simulink model "vco_test"  (Simulink 7.9)
settings: Solver=ode45  StartTime=0.0  StopTime=2  MaxStep=0.00001  RelTol=1e-3
values from neighbouring files (symbols this model uses):
  t_delay1 = t_delay1-0.1+0.2*rand(1)    [VCO_test.m]
  t_delay2 = t_delay2-0.1+0.2*rand(1)    [VCO_test.m]
  t_delay3 = t_delay3-0.1+0.2*rand(1)    [VCO_test.m]
libraries: dsparch4 x1, commsynccomp2 x1, commnoisgen2 x1, simulink x1, powerlib x1
settings Model: Creator=Administrator  LastModifiedBy=Administrator
settings DataIOCC: MaxDataPoints=1000000

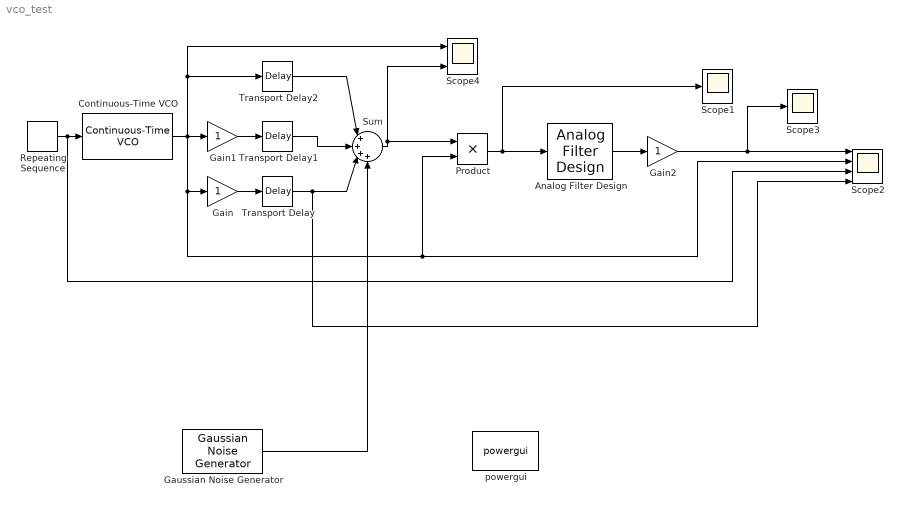
== system vco_test ==
  Analog Filter Design : dsparch4/Analog Filter Design  method=Butterworth  filttype=Lowpass  N=12  Wlo=2*3.14*25000  Whi=2*3.14*300  Rp=2  Rs=20
  Continuous-Time VCO : commsynccomp2/Continuous-Time VCO  Ac=1  Fc=100  Kc=10000  Ph=0
  Gain : Gain
  Gain1 : Gain
  Gain2 : Gain
  Gaussian Noise Generator : commnoisgen2/Gaussian Noise Generator  m=0  d=1  s=41  Ts=1  frameBased=off  sampPerFrame=1  orient=off  outDataType=double
  Product : Product  RndMeth=Zero
  Repeating Sequence : simulink/Sources/Repeating Sequence  rep_seq_t=[0 2]  rep_seq_y=[0 5]
  Scope1 : Scope
      settings: MaxDataPoints=10000001
  Scope2 : Scope  NumInputPorts=4
      settings: YMin=-5~-5~-5~-5  YMax=5~5~5~5  MaxDataPoints=131072  SampleInput=on  SampleTime=0.0001
  Scope3 : Scope
      settings: SaveName=ScopeData2  MaxDataPoints=10000001  SampleInput=on  SampleTime=0.00001
  Scope4 : Scope  NumInputPorts=2
      settings: YMin=-5~-5  YMax=5~5  SaveName=ScopeData3  MaxDataPoints=10000001  SampleInput=on  SampleTime=0.0001
  Sum : Sum  Inputs=|++++  SampleTime=0.0001
  Transport Delay : TransportDelay  DelayTime=t_delay3  BufferSize=5000000
  Transport Delay1 : TransportDelay  DelayTime=t_delay2  BufferSize=5000000
  Transport Delay2 : TransportDelay  DelayTime=t_delay1  BufferSize=5000000
  powergui : powerlib/powergui  Priority=1  SimulationMode=Discrete  SolverType=Tustin  SampleTime=1e-6  frequency=60  SPID=off  DisableSnubberDevices=off  DisableRonSwitches=off  DisableVfSwitches=off  SwTol=0  Interpol=off  DisplayEquations=off  FunctionMessages=off  frequencyindice=60  Pbase=100e6  ErrMax=1e-4  Iterations=50  UnitsV=kV  UnitsW=MW  echomessages=off  HookPort=off  EnableUseOfTLC=off  x0status=blocks  RestoreLinks=warning  ResistiveCurrentMeasurement=off  Ylog=off  Xlog=on  ShowGrid=off  save=off  variable=ZData  structure=ScopeData2  ZoomFFT=off  StartTime=0  cycles=2  DisplayStyle=1  fundamental=1  FreqAxis=off  MaxFrequency=25000  frequencyindicesteady=1  display=off  methode=off
  wires:
  Repeating Sequence/1 -> Scope2/3, Continuous-Time VCO/1
  Gain/1 -> Transport Delay/1
  Gain1/1 -> Transport Delay1/1
  Continuous-Time VCO/1 -> Gain1/1, Gain/1, Product/2, Scope2/2, Transport Delay2/1, Scope4/1
  Transport Delay2/1 -> Sum/1
  Transport Delay1/1 -> Sum/2
  Transport Delay/1 -> Sum/3, Scope2/4
  Sum/1 -> Scope4/2, Product/1
  Product/1 -> Scope1/1, Analog Filter Design/1
  Analog Filter Design/1 -> Gain2/1
  Gain2/1 -> Scope2/1, Scope3/1
  Gaussian Noise Generator/1 -> Sum/4
